simulink model "Expert_Online"  (R2021b)
settings: Solver=VariableStepAuto  StartTime=0.0  StopTime=10.0  RelTol=1e-3
model workspace (MAT data in the model file):
  a1 = 213
libraries: slpidlib x1
settings Model: Creator=yyfyyf  LastModifiedBy=yyfyyf

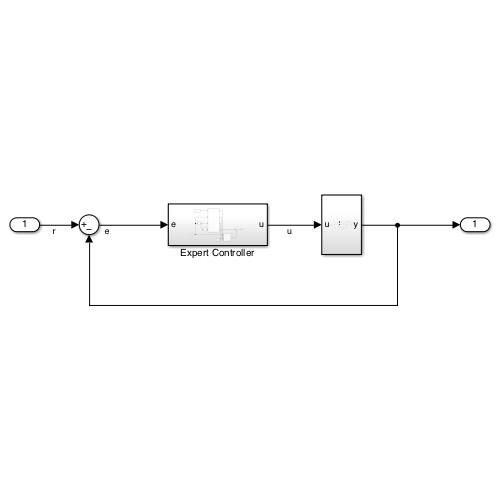
[thumbnail: Simulink's stored preview of the top-level diagram]
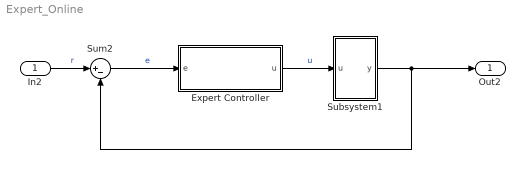
== system Expert_Online ==
  In2 : Inport  SampleTime=1e-3
  Expert Controller : Subsystem
  Subsystem1 : Subsystem
  Sum2 : Sum  Inputs=|+-
  Out2 : Outport
  wires:
  Expert Controller/1(u) -> Subsystem1/1(u)  "u"
  In2/1 -> Sum2/1  "r"
  Sum2/1 -> Expert Controller/1(e)  "e"
  Subsystem1/1(y) -> Sum2/2, Out2/1

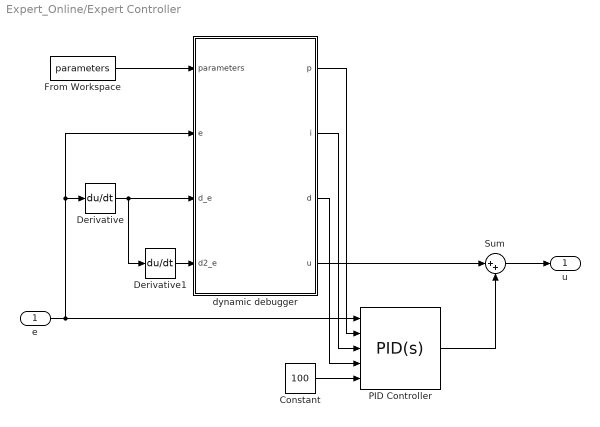
== system Expert_Online/Expert Controller ==
  e : Inport  SampleTime=0.00001
  Constant : Constant  Value=100
  Derivative : Derivative
  Derivative1 : Derivative
  From Workspace : FromWorkspace  VariableName=parameters
  PID Controller : slpidlib/PID Controller  Controller=PID  Form=Parallel  TimeDomain=Continuous-time  UseExternalTs=off  SampleTime=-1  IntegratorMethod=Forward Euler  FilterMethod=Forward Euler  ControllerParametersSource=external  P=1  I=1  D=0  UseFilter=on  N=100  TunerSelectOption=Transfer Function Based (PID Tuner App)  InitialConditionSource=internal  InitialConditionForIntegrator=0  InitialConditionForFilter=0  DifferentiatorICPrevScaledInput=0  ExternalReset=none  TrackingMode=off  Kt=1  LimitOutput=off  SatLimitsSource=internal  UpperSaturationLimit=inf  LowerSaturationLimit=-inf  LinearizeAsGain=on  AntiWindupMode=none  Kb=1  POutMin=[]  POutMax=[]  IOutMin=[]  IOutMax=[]  DOutMin=[]  DOutMax=[]  NOutMin=[]  NOutMax=[]  SumOutMin=[]  SumOutMax=[]  SaturationOutMin=[]  SaturationOutMax=[]  PParamMin=[]  PParamMax=[]  IParamMin=[]  IParamMax=[]  DParamMin=[]  DParamMax=[]  NParamMin=[]  NParamMax=[]  KbParamMin=[]  KbParamMax=[]  KtParamMin=[]  KtParamMax=[]  KbOutMin=[]  KbOutMax=[]  KtOutMin=[]  KtOutMax=[]  IntegratorOutMin=[]  IntegratorOutMax=[]  FilterOutMin=[]  FilterOutMax=[]  SumI1OutMin=[]  SumI1OutMax=[]  SumI2OutMin=[]  SumI2OutMax=[]  SumI3OutMin=[]  SumI3OutMax=[]  SumI4OutMin=[]  SumI4OutMax=[]  SumDOutMin=[]  SumDOutMax=[]  DifferentiatorOutMin=[]  DifferentiatorOutMax=[]  FilterDiffOutCoefMin=[]  FilterDiffOutCoefMax=[]  ReciprocalOutMin=[]  ReciprocalOutMax=[]  SumDenOutMin=[]  SumDenOutMax=[]  SumNumOutMin=[]  SumNumOutMax=[]  DivideOutMin=[]  DivideOutMax=[]  UdiffTsProdOutMin=[]  UdiffTsProdOutMax=[]  NTsProdOutMin=[]  NTsProdOutMax=[]  UintegralTsProdOutMin=[]  UintegralTsProdOutMax=[]  UngainTsProdOutMin=[]  UngainTsProdOutMax=[]  IntegratorContinuousStateAttributes=''  IntegratorStateMustResolveToSignalObject=off  IntegratorRTWStateStorageClass=Auto  FilterContinuousStateAttributes=''  FilterStateMustResolveToSignalObject=off  FilterRTWStateStorageClass=Auto  ParallelPVariant=ExternalParameters  IdealPVariant=Disabled  IVariant=ExternalParameters  DVariant=ExternalParameters  IntegratorVariant=Continuous  SatVariant=Disabled  AWVariant=Passthrough  PCopyVariant=Disabled  TRVariant=Disabled  FdbkBlocksVariant=Forward  IdealPFdbkVariant=Disabled  SatFdbkVariant=Disabled  DerivativeFilterVariant=ContFilter  NVariant=ExternalParameters  NCopyVariant=Disabled  FilterICVariant=InternalICsFilter  IntegratorICVariant=InternalICs  ExternalResetVariant=Disabled  TRSumVariant=Passthrough  SumFdbkVariant=Disabled  SumVariant=Sum_PID  TsampFilterVariant=InternalTs  TsampNgainVariant=Passthrough  TsampIntegralVariant=Passthrough  ExternalSaturationOutDataTypeStr=Inherit: Same as second input
  Sum : Sum  Inputs=|++
  dynamic debugger : MATLAB Function  TreatAsAtomicUnit=on
  u : Outport
  wires:
  e/1 -> dynamic debugger/2(e), Derivative/1, PID Controller/1
  Constant/1 -> PID Controller/5
  Sum/1 -> u/1
  dynamic debugger/1(p) -> PID Controller/2
  dynamic debugger/2(i) -> PID Controller/3
  dynamic debugger/3(d) -> PID Controller/4
  dynamic debugger/4(u) -> Sum/1
  PID Controller/1 -> Sum/2
  Derivative/1 -> Derivative1/1, dynamic debugger/3(d_e)
  From Workspace/1 -> dynamic debugger/1(parameters)
  Derivative1/1 -> dynamic debugger/4(d2_e)

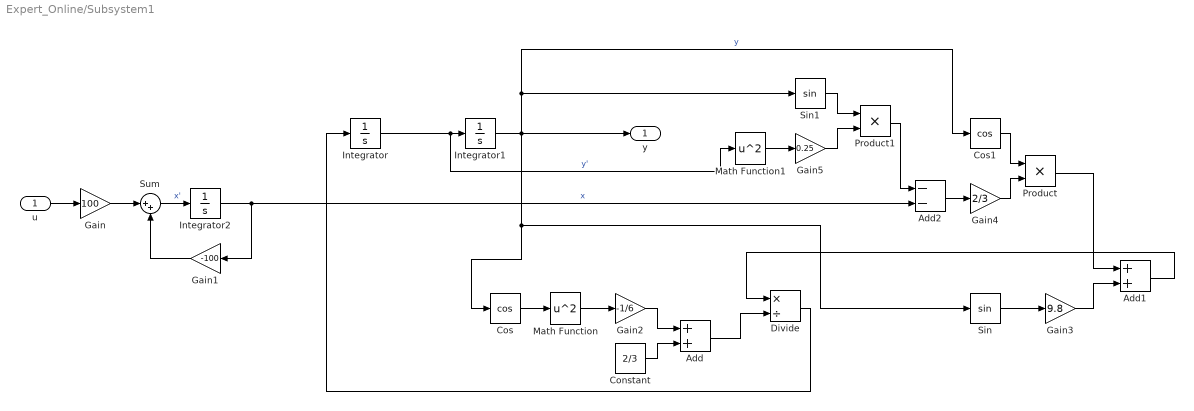
== system Expert_Online/Subsystem1 ==
  u : Inport
  Add : Sum
  Add1 : Sum
  Add2 : Sum  Inputs=--
  Constant : Constant  Value=2/3
  Cos : Trigonometry  Operator=cos
  Cos1 : Trigonometry  Operator=cos
  Divide : Product  Inputs=*/
  Gain : Gain  Gain=100
  Gain1 : Gain  Gain=-100
  Gain2 : Gain  Gain=-1/6
  Gain3 : Gain  Gain=9.8
  Gain4 : Gain  Gain=2/3
  Gain5 : Gain  Gain=0.25
  Integrator : Integrator
  Integrator1 : Integrator  InitialCondition=0.1
  Integrator2 : Integrator
  Math Function : Math  Operator=square  SaturateOnIntegerOverflow=on
  Math Function1 : Math  Operator=square  SaturateOnIntegerOverflow=on
  Product : Product
  Product1 : Product
  Sin : Trigonometry
  Sin1 : Trigonometry
  Sum : Sum  Inputs=|++
  y : Outport
  wires:
  Cos/1 -> Math Function/1
  Integrator1/1 -> Cos1/1, Sin1/1, y/1, Cos/1, Sin/1  "y"
  Constant/1 -> Add/2
  Add2/1 -> Gain4/1
  u/1 -> Gain/1
  Sum/1 -> Integrator2/1  "x'"
  Math Function1/1 -> Gain5/1
  Sin1/1 -> Product1/1
  Gain1/1 -> Sum/2
  Sin/1 -> Gain3/1
  Gain5/1 -> Product1/2
  Product1/1 -> Add2/1
  Product/1 -> Add1/1
  Add/1 -> Divide/2
  Add1/1 -> Divide/1
  Integrator/1 -> Math Function1/1, Integrator1/1  "y'"
  Gain/1 -> Sum/1
  Gain2/1 -> Add/1
  Divide/1 -> Integrator/1
  Integrator2/1 -> Gain1/1, Add2/2  "x"
  Cos1/1 -> Product/1
  Gain4/1 -> Product/2
  Math Function/1 -> Gain2/1
  Gain3/1 -> Add1/2

== matlab function Expert_Online/Expert Controller/dynamic debugger ==
  data: parameters input; e input; p output; i output; d output; u output; d_e input; d2_e input
function [p, i, d, u] = dynamic(parameters, e, d_e, d2_e)


p_0 = parameters(1);
i_0 = parameters(2);
d_0 = parameters(3);

p_1 = parameters(4);
i_1 = parameters(5);
d_1 = parameters(6);

p_2 = parameters(7);
i_2 = parameters(8);
d_2 = parameters(9);

u = 0;
if e * d_e < 0
    if d2_e < 0
     
        p = p_0;
        i = i_0;
        d = d_0;
    else
      
        p = p_1;
        i = i_1;
        d = d_1;
    end
else

    p = p_2;
    i = i_2;
    d = d_2;
end   

end
